simulink model "ProtectionSystem"  (R2020a)
settings: Solver=VariableStepAuto  StartTime=0.0  StopTime=10.0  RelTol=1e-3
undefined symbols (not defined in the file or in its folder): Accelerationmax, Accelerationmin, IDCmax, IDCmin, Iphasepeakmax, Risetimemax, Speedmax, Stalltimemax, Temperaturemax, VDCmax, VDCmin, VDCrated
libraries: simulink x28, powerlib_meascontrol x2
settings Model: Creator=Sony  LastModifiedBy=Sony

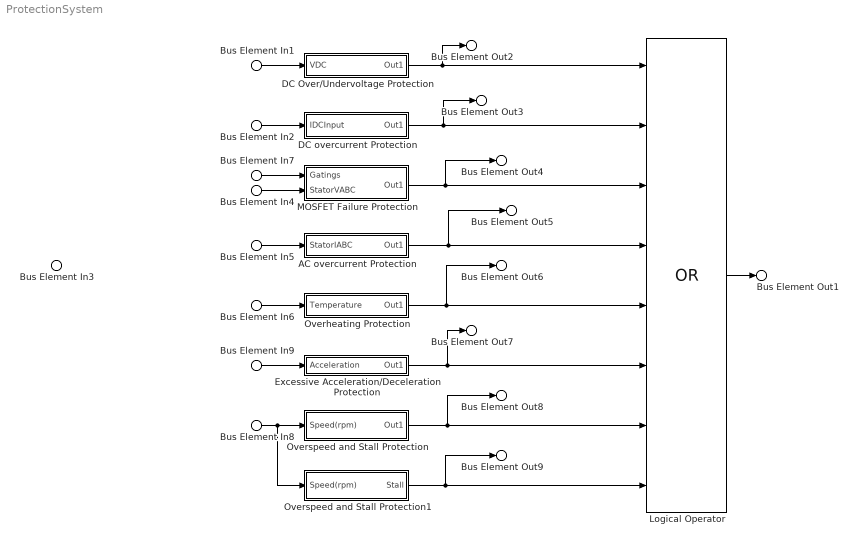
== system ProtectionSystem ==
  Bus Element In1 : Inport  PortName=Sampled DC Input Voltage VDC
  Bus Element In2 : Inport  Port=2  PortName=Sampled DC Input Current IDC
  Bus Element In4 : Inport  Port=3  PortName=Sampled Stator VABC
  Bus Element In5 : Inport  Port=4  PortName=Sampled Stator IABC
  Bus Element In3 : Inport  Port=5  PortName=Sampled HALL Signals HABC
  Bus Element In6 : Inport  Port=6  PortName=Sampled Temperature
  Bus Element In8 : Inport  Port=7  PortName=Sampled Speed (rpm)
  Bus Element In7 : Inport  Port=8  PortName=Sampled Inverter Gatings
  Bus Element In9 : Inport  Port=9  PortName=Sampled Acceleration
  AC overcurrent Protection : Subsystem
  DC Over/Undervoltage Protection : Subsystem
  DC overcurrent Protection : Subsystem
  Excessive Acceleration/Deceleration Protection : Subsystem
  Logical Operator : Logic  Operator=OR  Inputs=8  AllPortsSameDT=off  OutDataTypeStr=boolean
  MOSFET Failure Protection : Subsystem
  Overheating Protection : Subsystem
  Overspeed and Stall Protection : Subsystem
  Overspeed and Stall Protection1 : Subsystem
  Bus Element Out1 : Outport  PortName=Shutdown
  Bus Element Out2 : Outport  Port=2  PortName=Input DC over/ under-voltage
  Bus Element Out3 : Outport  Port=3  PortName=Input DC over-current
  Bus Element Out4 : Outport  Port=4  PortName=MOSFET failure
  Bus Element Out5 : Outport  Port=5  PortName=AC overcurrent
  Bus Element Out6 : Outport  Port=6  PortName=Overheating
  Bus Element Out7 : Outport  Port=7  PortName=Excessive acceleration/ deceleration
  Bus Element Out8 : Outport  Port=8  PortName=Overspeed
  Bus Element Out9 : Outport  Port=9  PortName=Stall
  wires:
  Overspeed and Stall Protection/1(Out1) -> Bus Element Out8/1, Logical Operator/7
  Bus Element In6/1 -> Overheating Protection/1(Temperature)
  Bus Element In8/1 -> Overspeed and Stall Protection1/1(Speed(rpm)), Overspeed and Stall Protection/1(Speed(rpm))
  Bus Element In9/1 -> Excessive Acceleration/Deceleration Protection/1(Acceleration)
  Bus Element In4/1 -> MOSFET Failure Protection/2(StatorVABC)
  Bus Element In5/1 -> AC overcurrent Protection/1(StatorIABC)
  Bus Element In1/1 -> DC Over/Undervoltage Protection/1(VDC)
  Bus Element In2/1 -> DC overcurrent Protection/1(IDCInput)
  Excessive Acceleration/Deceleration Protection/1(Out1) -> Bus Element Out7/1, Logical Operator/6
  MOSFET Failure Protection/1(Out1) -> Bus Element Out4/1, Logical Operator/3
  Logical Operator/1 -> Bus Element Out1/1
  Bus Element In7/1 -> MOSFET Failure Protection/1(Gatings)
  AC overcurrent Protection/1(Out1) -> Bus Element Out5/1, Logical Operator/4
  DC overcurrent Protection/1(Out1) -> Bus Element Out3/1, Logical Operator/2
  Overheating Protection/1(Out1) -> Bus Element Out6/1, Logical Operator/5
  DC Over/Undervoltage Protection/1(Out1) -> Logical Operator/1, Bus Element Out2/1
  Overspeed and Stall Protection1/1(Stall) -> Bus Element Out9/1, Logical Operator/8

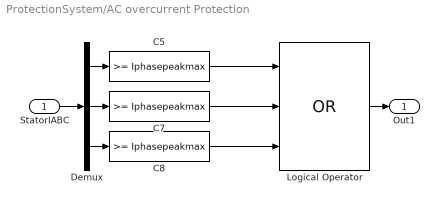
== system ProtectionSystem/AC overcurrent Protection ==
  StatorIABC : Inport
  C5 : simulink/Logic and Bit Operations/Compare To Constant  relop=>=  const=Iphasepeakmax  OutDataTypeStr=boolean
  C7 : simulink/Logic and Bit Operations/Compare To Constant  relop=>=  const=Iphasepeakmax  OutDataTypeStr=boolean
  C8 : simulink/Logic and Bit Operations/Compare To Constant  relop=>=  const=Iphasepeakmax  OutDataTypeStr=boolean
  Demux : Demux  Outputs=3
  Logical Operator : Logic  Operator=OR  Inputs=3  AllPortsSameDT=off  OutDataTypeStr=boolean
  Out1 : Outport
  wires:
  C5/1 -> Logical Operator/1
  C8/1 -> Logical Operator/3
  C7/1 -> Logical Operator/2
  StatorIABC/1 -> Demux/1
  Demux/2 -> C7/1
  Demux/3 -> C8/1
  Demux/1 -> C5/1
  Logical Operator/1 -> Out1/1

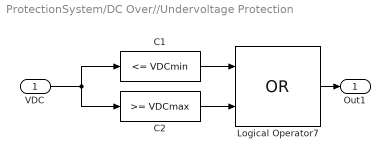
== system ProtectionSystem/DC Over//Undervoltage Protection ==
  VDC : Inport
  C1 : simulink/Logic and Bit Operations/Compare To Constant  relop=<=  const=VDCmin  OutDataTypeStr=boolean
  C2 : simulink/Logic and Bit Operations/Compare To Constant  relop=>=  const=VDCmax  OutDataTypeStr=boolean
  Logical Operator7 : Logic  Operator=OR  AllPortsSameDT=off  OutDataTypeStr=boolean
  Out1 : Outport
  wires:
  VDC/1 -> C2/1, C1/1
  Logical Operator7/1 -> Out1/1
  C1/1 -> Logical Operator7/1
  C2/1 -> Logical Operator7/2

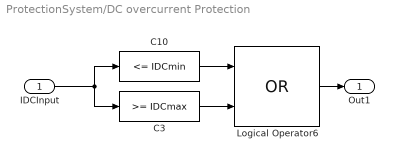
== system ProtectionSystem/DC overcurrent Protection ==
  IDCInput : Inport
  C10 : simulink/Logic and Bit Operations/Compare To Constant  relop=<=  const=IDCmin  OutDataTypeStr=boolean
  C3 : simulink/Logic and Bit Operations/Compare To Constant  relop=>=  const=IDCmax  OutDataTypeStr=boolean
  Logical Operator6 : Logic  Operator=OR  AllPortsSameDT=off  OutDataTypeStr=boolean
  Out1 : Outport
  wires:
  C10/1 -> Logical Operator6/1
  C3/1 -> Logical Operator6/2
  IDCInput/1 -> C3/1, C10/1
  Logical Operator6/1 -> Out1/1

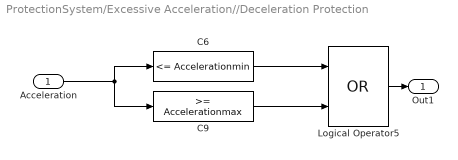
== system ProtectionSystem/Excessive Acceleration//Deceleration Protection ==
  Acceleration : Inport
  C6 : simulink/Logic and Bit Operations/Compare To Constant  relop=<=  const=Accelerationmin  OutDataTypeStr=boolean
  C9 : simulink/Logic and Bit Operations/Compare To Constant  relop=>=  const=Accelerationmax  OutDataTypeStr=boolean
  Logical Operator5 : Logic  Operator=OR  AllPortsSameDT=off  OutDataTypeStr=boolean
  Out1 : Outport
  wires:
  C9/1 -> Logical Operator5/2
  Acceleration/1 -> C9/1, C6/1
  Logical Operator5/1 -> Out1/1
  C6/1 -> Logical Operator5/1

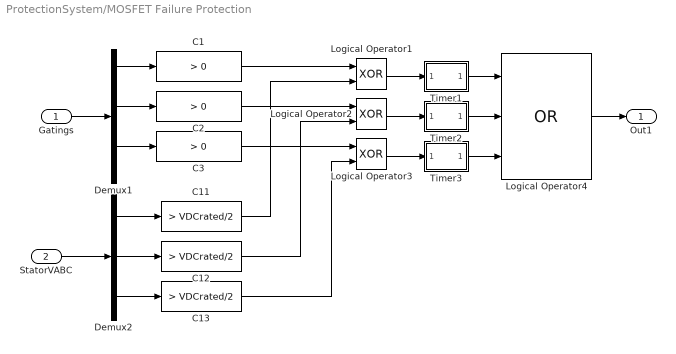
== system ProtectionSystem/MOSFET Failure Protection ==
  Gatings : Inport
  StatorVABC : Inport  Port=2
  C1 : simulink/Logic and Bit Operations/Compare To Constant  relop=>  const=0  OutDataTypeStr=boolean
  C11 : simulink/Logic and Bit Operations/Compare To Constant  relop=>  const=VDCrated/2  OutDataTypeStr=boolean
  C12 : simulink/Logic and Bit Operations/Compare To Constant  relop=>  const=VDCrated/2  OutDataTypeStr=boolean
  C13 : simulink/Logic and Bit Operations/Compare To Constant  relop=>  const=VDCrated/2  OutDataTypeStr=boolean
  C2 : simulink/Logic and Bit Operations/Compare To Constant  relop=>  const=0  OutDataTypeStr=boolean
  C3 : simulink/Logic and Bit Operations/Compare To Constant  relop=>  const=0  OutDataTypeStr=boolean
  Demux1 : Demux  Outputs=6
  Demux2 : Demux  Outputs=3
  Logical Operator1 : Logic  Operator=XOR  AllPortsSameDT=off  OutDataTypeStr=boolean
  Logical Operator2 : Logic  Operator=XOR  AllPortsSameDT=off  OutDataTypeStr=boolean
  Logical Operator3 : Logic  Operator=XOR  AllPortsSameDT=off  OutDataTypeStr=boolean
  Logical Operator4 : Logic  Operator=OR  Inputs=3  AllPortsSameDT=off  OutDataTypeStr=boolean
  Timer1 : Subsystem
  Timer2 : Subsystem
  Timer3 : Subsystem
  Out1 : Outport
  wires:
  Logical Operator3/1 -> Timer3/1(In1)
  Demux2/3 -> C13/1
  Logical Operator2/1 -> Timer2/1(In1)
  StatorVABC/1 -> Demux2/1
  Gatings/1 -> Demux1/1
  Demux1/3 -> C2/1
  Demux1/1 -> C1/1
  Demux1/5 -> C3/1
  Demux2/1 -> C11/1
  C13/1 -> Logical Operator3/2
  C11/1 -> Logical Operator1/2
  Demux2/2 -> C12/1
  Logical Operator1/1 -> Timer1/1(In1)
  C12/1 -> Logical Operator2/2
  Logical Operator4/1 -> Out1/1
  C1/1 -> Logical Operator1/1
  C2/1 -> Logical Operator2/1
  C3/1 -> Logical Operator3/1
  Timer1/1(Out1) -> Logical Operator4/1
  Timer2/1(Out1) -> Logical Operator4/2
  Timer3/1(Out1) -> Logical Operator4/3

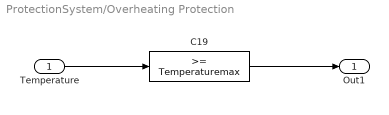
== system ProtectionSystem/Overheating Protection ==
  Temperature : Inport
  C19 : simulink/Logic and Bit Operations/Compare To Constant  relop=>=  const=Temperaturemax  OutDataTypeStr=boolean
  Out1 : Outport
  wires:
  Temperature/1 -> C19/1
  C19/1 -> Out1/1

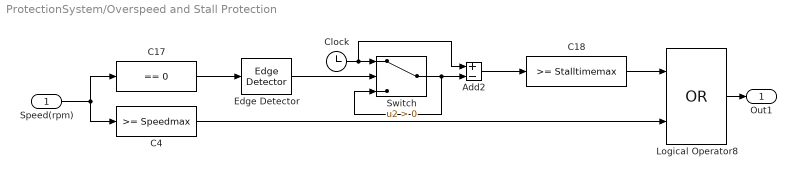
== system ProtectionSystem/Overspeed and Stall Protection ==
  Speed(rpm) : Inport
  Add2 : Sum  Inputs=+-
  C17 : simulink/Logic and Bit Operations/Compare To Constant  relop===  const=0  OutDataTypeStr=boolean
  C18 : simulink/Logic and Bit Operations/Compare To Constant  relop=>=  const=Stalltimemax  OutDataTypeStr=boolean
  C4 : simulink/Logic and Bit Operations/Compare To Constant  relop=>=  const=Speedmax  OutDataTypeStr=boolean
  Clock : Clock
      settings: Decimation=1000000
  Edge Detector : powerlib_meascontrol/Logic/Edge Detector  model=Rising  ic=0  Ts=0
      settings: SourceProductBaseCode=PS
  Logical Operator8 : Logic  Operator=OR  AllPortsSameDT=off  OutDataTypeStr=boolean
  Switch : Switch  Criteria=u2 > Threshold
  Out1 : Outport
  wires:
  C18/1 -> Logical Operator8/1
  Logical Operator8/1 -> Out1/1
  Speed(rpm)/1 -> C4/1, C17/1
  Add2/1 -> C18/1
  C17/1 -> Edge Detector/1
  Switch/1 -> Switch/3, Add2/2
  Edge Detector/1 -> Switch/2
  Clock/1 -> Add2/1, Switch/1
  C4/1 -> Logical Operator8/2

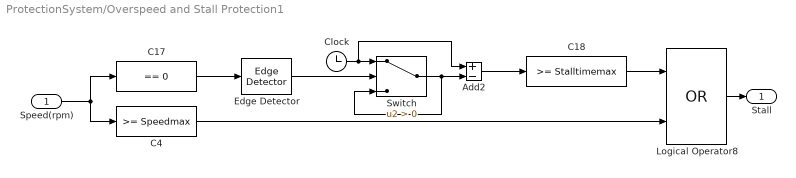
== system ProtectionSystem/Overspeed and Stall Protection1 ==
  Speed(rpm) : Inport
  Add2 : Sum  Inputs=+-
  C17 : simulink/Logic and Bit Operations/Compare To Constant  relop===  const=0  OutDataTypeStr=boolean
  C18 : simulink/Logic and Bit Operations/Compare To Constant  relop=>=  const=Stalltimemax  OutDataTypeStr=boolean
  C4 : simulink/Logic and Bit Operations/Compare To Constant  relop=>=  const=Speedmax  OutDataTypeStr=boolean
  Clock : Clock
      settings: Decimation=1000000
  Edge Detector : powerlib_meascontrol/Logic/Edge Detector  model=Rising  ic=0  Ts=0
      settings: SourceProductBaseCode=PS
  Logical Operator8 : Logic  Operator=OR  AllPortsSameDT=off  OutDataTypeStr=boolean
  Switch : Switch  Criteria=u2 > Threshold
  Stall : Outport
  wires:
  C18/1 -> Logical Operator8/1
  Logical Operator8/1 -> Stall/1
  Speed(rpm)/1 -> C4/1, C17/1
  Add2/1 -> C18/1
  C17/1 -> Edge Detector/1
  Switch/1 -> Switch/3, Add2/2
  Edge Detector/1 -> Switch/2
  Clock/1 -> Add2/1, Switch/1
  C4/1 -> Logical Operator8/2

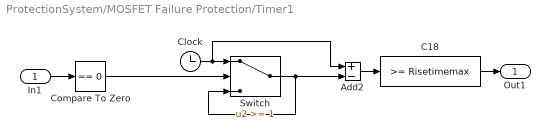
== system ProtectionSystem/MOSFET Failure Protection/Timer1 ==
  In1 : Inport
  Add2 : Sum  Inputs=+-
  C18 : simulink/Logic and Bit Operations/Compare To Constant  relop=>=  const=Risetimemax  OutDataTypeStr=boolean
  Clock : Clock
      settings: Decimation=1000000
  Compare To Zero : simulink/Logic and Bit Operations/Compare To Zero  relop===  OutDataTypeStr=boolean
  Switch : Switch  Threshold=1
  Out1 : Outport
  wires:
  Add2/1 -> C18/1
  In1/1 -> Compare To Zero/1
  Compare To Zero/1 -> Switch/2
  Switch/1 -> Switch/3, Add2/2
  Clock/1 -> Add2/1, Switch/1
  C18/1 -> Out1/1

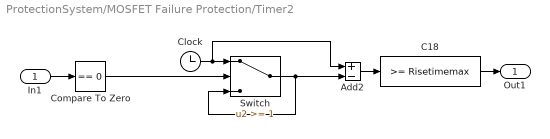
== system ProtectionSystem/MOSFET Failure Protection/Timer2 ==
  In1 : Inport
  Add2 : Sum  Inputs=+-
  C18 : simulink/Logic and Bit Operations/Compare To Constant  relop=>=  const=Risetimemax  OutDataTypeStr=boolean
  Clock : Clock
      settings: Decimation=1000000
  Compare To Zero : simulink/Logic and Bit Operations/Compare To Zero  relop===  OutDataTypeStr=boolean
  Switch : Switch  Threshold=1
  Out1 : Outport
  wires:
  Add2/1 -> C18/1
  In1/1 -> Compare To Zero/1
  Compare To Zero/1 -> Switch/2
  Switch/1 -> Switch/3, Add2/2
  Clock/1 -> Add2/1, Switch/1
  C18/1 -> Out1/1

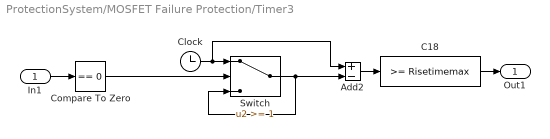
== system ProtectionSystem/MOSFET Failure Protection/Timer3 ==
  In1 : Inport
  Add2 : Sum  Inputs=+-
  C18 : simulink/Logic and Bit Operations/Compare To Constant  relop=>=  const=Risetimemax  OutDataTypeStr=boolean
  Clock : Clock
      settings: Decimation=1000000
  Compare To Zero : simulink/Logic and Bit Operations/Compare To Zero  relop===  OutDataTypeStr=boolean
  Switch : Switch  Threshold=1
  Out1 : Outport
  wires:
  Add2/1 -> C18/1
  In1/1 -> Compare To Zero/1
  Compare To Zero/1 -> Switch/2
  Switch/1 -> Switch/3, Add2/2
  Clock/1 -> Add2/1, Switch/1
  C18/1 -> Out1/1
